simulink model "Indirect_field_oriented_control"  (R2021a)
settings: Solver=VariableStepAuto  StartTime=0.0  StopTime=10.0  RelTol=1e-3
undefined symbols (not defined in the file): magnitude
settings Model: Creator=Mehra  LastModifiedBy=Mehra

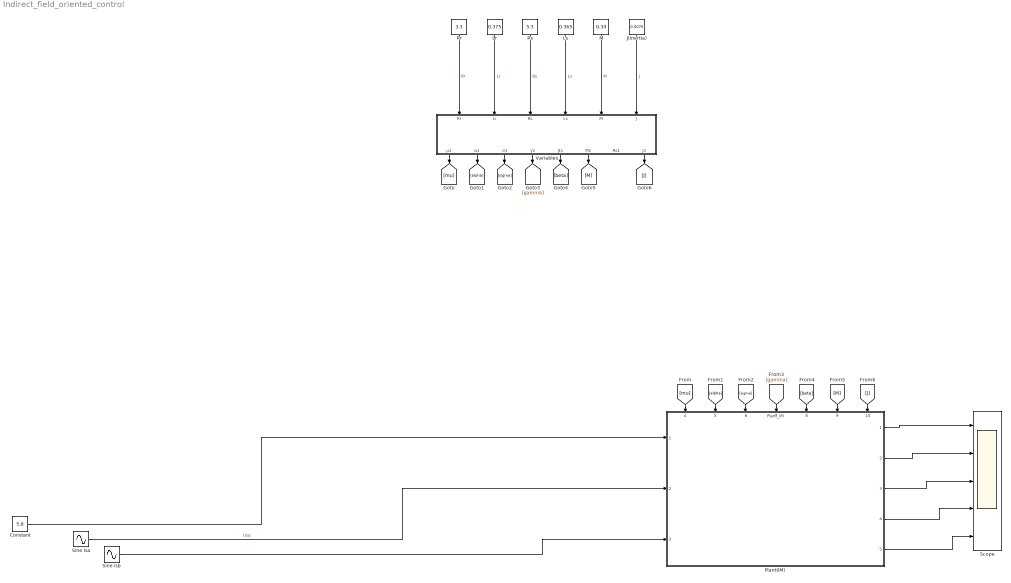
== system Indirect_field_oriented_control ==
  Constant : Constant  Value=5.8
  J(inertia) : Constant  Value=0.0075
  Lr : Constant  Value=0.375
  Ls : Constant  Value=0.365
  M : Constant  Value=0.34
  Plant(IM) : ModelReference  ModelNameDialog=Plant_IM  SimulationMode=Normal  ModelReferenceVersion=1.20
      settings: PortSchema="{\"entries\":[{\"content\":{\"sides\":[{\"content\":{\"connectorIds\":[\"In1\",\"In2\",\"In3\"]},\"type\":\"ConnectorPlacement.EquallySpacedRectSide\",\"uuid\":\"c1ced4ac-9292-447b-a16b-48862d3db151\"},{\"content\":{\"connectorIds\":[\"Out1\",\"Out2\",\"Out3\",\"Out4\",\"Out5\"],\"side\":\"RIGHT\"},\"type\":\"ConnectorPlacement.EquallySpacedRectSide\",\"uuid\":\"13a72579-fb39-4c86-8f38-f8272c138e74\"},{\"content\":{\"connectorIds\":[\"In4\",\"In5\",\"In6\",\"In7\",\"In8\",\"In9\",\"In10\"],\"side\":\"TOP\"},\"type\":\"ConnectorPlacement.EquallySpacedRectSide\",\"uuid\":\"7112169d-3c72-435f-89ee-d1fe7807fab2\"}]},\"type\":\"ConnectorPlacement.EquallySpacedConnector\",\"uuid\":\"c43df563-9598-43b0-9064-e7550f78106e\"}],\"packageUris\":[\"http://schema.mathworks.com/mf0/Connector/R2020b\"],\"version\":\"1.0\"}"
  Rr : Constant  Value=3.3
  Rs : Constant  Value=5.3
  Scope : Scope  NumInputPorts=5
  Sine isa : Sin  Amplitude=5  Frequency=60  Phase=1.15  SampleTime=0
  Sine isb : Sin  Amplitude=5  Frequency=60  SampleTime=0
  Variables : Subsystem
  wires:
  Plant(IM)/1 -> Scope/1
  Plant(IM)/2 -> Scope/2
  Plant(IM)/3 -> Scope/3
  Sine isb/1 -> Plant(IM)/3
  Sine isa/1 -> Plant(IM)/2  "Usa"
  Constant/1 -> Plant(IM)/1
  J(inertia)/1 -> Variables/6(J)  "J"
  M/1 -> Variables/5(M)  "M"
  Rr/1 -> Variables/1(Rr)  "Rr"
  Lr/1 -> Variables/2(Lr)  "Lr"
  Rs/1 -> Variables/3(Rs)  "Rs"
  Ls/1 -> Variables/4(Ls)  "Ls"
  Plant(IM)/5 -> Scope/5
  Plant(IM)/4 -> Scope/4
  [mu] -> Plant(IM)/4
  Variables/1(µ1) -> [mu]
  [alpha] -> Plant(IM)/5
  [sigma] -> Plant(IM)/6
  [gamma] -> Plant(IM)/7
  [beta] -> Plant(IM)/8
  [M] -> Plant(IM)/9
  [J] -> Plant(IM)/10
  Variables/2(α1) -> [alpha]
  Variables/3(σ1) -> [sigma]
  Variables/4(γ1) -> [gamma]
  Variables/5(β1) -> [beta]
  Variables/6(M1) -> [M]
  Variables/8(J1) -> [J]

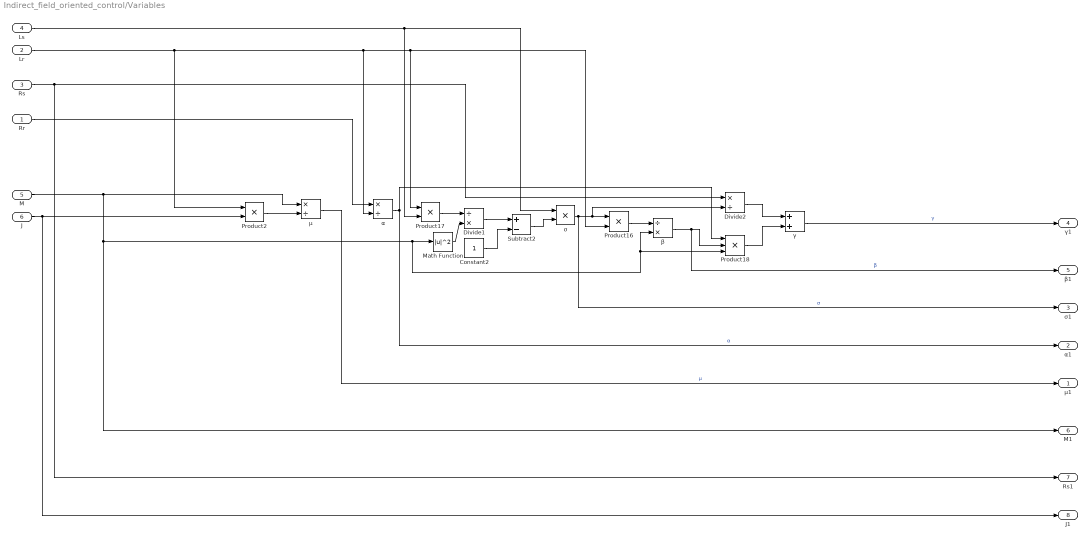
== system Indirect_field_oriented_control/Variables ==
  Rr : Inport
  Lr : Inport  Port=2
  Rs : Inport  Port=3
  Ls : Inport  Port=4
  M : Inport  Port=5
  J : Inport  Port=6
  Constant2 : Constant
  Divide1 : Product  Inputs=/*
  Divide2 : Product  Inputs=*/
  Math Function : Math  Operator=magnitude^2  SaturateOnIntegerOverflow=on
  Product16 : Product
  Product17 : Product
  Product18 : Product  Inputs=3
  Product2 : Product
  Subtract2 : Sum  Inputs=+-
  µ : Product  Inputs=*/
  α : Product  Inputs=*/
  β : Product  Inputs=/*
  γ : Sum
  σ : Product
  µ1 : Outport
  α1 : Outport  Port=2
  σ1 : Outport  Port=3
  γ1 : Outport  Port=4
  β1 : Outport  Port=5
  M1 : Outport  Port=6
  Rs1 : Outport  Port=7
  J1 : Outport  Port=8
  wires:
  Divide1/1 -> Subtract2/1
  Math Function/1 -> Divide1/2
  Constant2/1 -> Subtract2/2
  Divide2/1 -> γ/1
  Lr/1 -> Product17/1, Product16/2, α/2, Product2/1
  σ/1 -> σ1/1, Product16/1, Divide2/2  "σ"
  Product2/1 -> µ/2
  β/1 -> β1/1, Product18/2  "β"
  Product17/1 -> Divide1/1
  Product16/1 -> β/1
  Subtract2/1 -> σ/2
  J/1 -> J1/1, Product2/2
  M/1 -> M1/1, Product18/3, β/2, Math Function/1, µ/1
  Ls/1 -> Product17/2, σ/1
  α/1 -> α1/1, Product18/1  "α"
  Product18/1 -> γ/2
  γ/1 -> γ1/1  "γ"
  Rr/1 -> α/1
  µ/1 -> µ1/1  "µ"
  Rs/1 -> Rs1/1, Divide2/1
